simulink model "sm_import_robot_stepfiles"  (R2018b)
settings: Solver=FixedStepAuto  StartTime=0.0  StopTime=50  RelTol=1e-3  EnableMultiTasking=on
undefined symbols (not defined in the file): sigbuilder_block, X, Y, Z
libraries: sm_lib x58, fl_lib x41, nesl_utility x23, Multibody_Multiphysics_Lib x6, elec_lib x3, dspindex x3, arduinolib x2
(part 3 of 3)

== system sm_import_robot_stepfiles/Robot/Gripper/Right Second Finger Link ==
  Base Transform : sm_lib/Frames and Transforms/Rigid Transform  TranslationMethod=Cartesian  TranslationStandardOffset=0  TranslationLengthUnit=cm  TranslationStandardAxis=+Z  TranslationCartesianOffset=[2.1844 -0.91801024484276539 0]  TranslationROffset=0  TranslationROffsetUnits=m  TranslationZOffset=0  TranslationZOffsetUnits=m  TranslationThetaOffset=0  TranslationThetaOffsetUnits=deg  RotationMethod=ArbitraryAxis  RotationAngleUnits=deg  RotationStandardAxis=+Z  RotationAngle=120  RotationArbitraryAxis=[-1 -1 -1]  FollAlignAxisA=+X  BaseAlignAxisA=+Y  FollAlignAxisB=+Y  BaseAlignAxisB=+Z  RotationSequenceAxes=FollowerAxes  RotationSequence=XYX  RotationSequenceAngles=[0 0 0]  RotationSequenceAnglesUnits=deg  RotationMatrix=[1 0 0; 0 1 0; 0 0 1]
  Follower Transform : sm_lib/Frames and Transforms/Rigid Transform  TranslationMethod=Cartesian  TranslationStandardOffset=0  TranslationLengthUnit=cm  TranslationStandardAxis=+Z  TranslationCartesianOffset=[0 0.61321024484276621 0]  TranslationROffset=0  TranslationROffsetUnits=m  TranslationZOffset=0  TranslationZOffsetUnits=m  TranslationThetaOffset=0  TranslationThetaOffsetUnits=deg  RotationMethod=ArbitraryAxis  RotationAngleUnits=deg  RotationStandardAxis=+Z  RotationAngle=120  RotationArbitraryAxis=[1 -1 1]  FollAlignAxisA=+X  BaseAlignAxisA=+Y  FollAlignAxisB=+Y  BaseAlignAxisB=+Z  RotationSequenceAxes=FollowerAxes  RotationSequence=XYX  RotationSequenceAngles=[0 0 0]  RotationSequenceAnglesUnits=deg  RotationMatrix=[1 0 0; 0 1 0; 0 0 1]
  Solid : sm_lib/Body Elements/Solid  InertiaType=CalculateFromGeometry  Mass=0.005347817964666832  MassUnits=kg  CenterOfMass=[1.3095387695944416 0 0]  CenterOfMassUnits=cm  MomentsOfInertia=[0.00062632050801362594 0.0042402045040431545 0.0044495724115703027]  MomentsOfInertiaUnits=kg*cm^2  ProductsOfInertia=[0 0 0]  ProductsOfInertiaUnits=kg*cm^2  BasedOnType=Mass  Density=1000  DensityUnits=kg/(m^3)  DoExposeReferenceFrame=on  SerializedFrames=<Frames/>  GraphicType=FromGeometry  MarkerShape=Sphere  MarkerSize=10  MarkerSizeUnits=m  GraphicVisPropType=SimpleVisualProperties  GraphicDiffuseColor=[1 0 0]  GraphicSpecularColor=[0.5 0.5 0.5 1.0]  GraphicAmbientColor=[0.15 0.15 0.15 1.0]  GraphicEmissiveColor=[0.0 0.0 0.0 1.0]  GraphicShininess=75  GraphicOpacity=1  GeometryShape=FromFile  RectangleSize=[1 1]  RectangleSizeUnits=m  BrickDimensions=[1 1 1]  BrickDimensionUnits=m  CylinderRadius=1  CylinderRadiusUnits=m  CylinderLength=1  CylinderLengthUnits=m  SphereRadius=1  SphereRadiusUnits=m  EllipsoidRadii=[1 1 1]  EllipsoidRadiiUnits=m  ExtrusionCrossSection=[1 1; -1 1; -1 -1; 1 -1]  ExtrusionCrossSectionUnits=m  ExtrusionLength=1  ExtrusionLengthUnits=m  PolygonNumSides=3  PolygonOuterRadius=1  PolygonOuterRadiusUnits=m  ExtGeomFileType=STEP  ExtGeomFileName=sm_srobot_secondfingerlink.step  ExtGeomFileUnits=cm  RevolutionCrossSection=[1 1; 1 -1; 2 -1; 2 1]  RevolutionCrossSectionUnits=m  RevolutionExtent=Full  RevolutionAngle=180  RevolutionAngleUnits=deg
  B : PMIOPort  Side=Left
  F : PMIOPort  Port=2  Side=Right
  connections:
  Solid/RConn1 -- Follower Transform/LConn1 -- Base Transform/LConn1
  Base Transform/RConn1 -- B/RConn1
  Follower Transform/RConn1 -- F/RConn1

== system sm_import_robot_stepfiles/Robot/Gripper Actuation/Gripper Motion ==
  Demux : Demux  Tag=STV Demux  Outputs=1
  FromWs : FromWorkspace  Tag=STV FromWs  VariableName=tuvar  SampleTime=0
      SigBuilderData=|
      | common.afterFinalStr = 'Extrapolate'
      | common.sampleTime = 0
      | dataSet.timeRange = [0 20]
      | dataSet.name = 'Motion'
      | sbobj.Groups.Name = 'Motion'
      | sbobj.Groups.Signals.Name = 'GA'
      | sbobj.Groups.Signals.XData = [0 2.5 4.5 5.5 7.5 12.5 14.5 15.5 17.5 20]
      | sbobj.Groups.Signals.YData = [0 0 0.5 0 0 0 -0.2 -0.2 0 0]
      | sbobj.Groups.TimeRange = [0 20]
  GA : Outport  Tag=STV Outport
  wires:
  Demux/1 -> GA/1
  FromWs/1 -> Demux/1

== system sm_import_robot_stepfiles/Robot/DC Motor1/Counter1/counterA ==
  In1 : Inport
  In2 : Inport  Port=2
  Trigger : TriggerPort  TriggerType=either  VariantControl=Variant  PortDimensions=1
  Add : Sum
  Constant : Constant  SampleTime=-1
  Constant1 : Constant  Value=-1  SampleTime=-1
  Logical Operator : Logic  Operator=XOR  AllPortsSameDT=off  OutDataTypeStr=boolean
  Memory : Memory  InheritSampleTime=on
  Switch : Switch  Criteria=u2 > Threshold
  Out1 : Outport
  wires:
  Constant1/1 -> Switch/3
  Constant/1 -> Switch/1
  Switch/1 -> Add/1
  Logical Operator/1 -> Switch/2
  In2/1 -> Logical Operator/2  "B"
  In1/1 -> Logical Operator/1  "A"
  Add/1 -> Memory/1, Out1/1
  Memory/1 -> Add/2

== system sm_import_robot_stepfiles/Robot/DC Motor1/Counter1/counterB ==
  In1 : Inport
  In2 : Inport  Port=2
  Trigger : TriggerPort  TriggerType=either  VariantControl=Variant  PortDimensions=1
  Add : Sum
  Constant : Constant  Value=-1  SampleTime=-1
  Constant1 : Constant  SampleTime=-1
  Logical Operator : Logic  Operator=XOR  AllPortsSameDT=off  OutDataTypeStr=boolean
  Memory : Memory  InheritSampleTime=on
  Switch : Switch  Criteria=u2 > Threshold
  Out1 : Outport
  wires:
  Memory/1 -> Add/2
  Add/1 -> Out1/1, Memory/1
  In1/1 -> Logical Operator/1  "A"
  In2/1 -> Logical Operator/2  "B"
  Logical Operator/1 -> Switch/2
  Switch/1 -> Add/1
  Constant/1 -> Switch/1
  Constant1/1 -> Switch/3

== system sm_import_robot_stepfiles/Robot/DC Motor2/Counter1/counterA ==
  In1 : Inport
  In2 : Inport  Port=2
  Trigger : TriggerPort  TriggerType=either  VariantControl=Variant  PortDimensions=1
  Add : Sum
  Constant : Constant  SampleTime=-1
  Constant1 : Constant  Value=-1  SampleTime=-1
  Logical Operator : Logic  Operator=XOR  AllPortsSameDT=off  OutDataTypeStr=boolean
  Memory : Memory  InheritSampleTime=on
  Switch : Switch  Criteria=u2 > Threshold
  Out1 : Outport
  wires:
  Memory/1 -> Add/2
  Add/1 -> Out1/1, Memory/1
  In1/1 -> Logical Operator/1  "A"
  In2/1 -> Logical Operator/2  "B"
  Logical Operator/1 -> Switch/2
  Switch/1 -> Add/1
  Constant/1 -> Switch/1
  Constant1/1 -> Switch/3

== system sm_import_robot_stepfiles/Robot/DC Motor2/Counter1/counterB ==
  In1 : Inport
  In2 : Inport  Port=2
  Trigger : TriggerPort  TriggerType=either  VariantControl=Variant  PortDimensions=1
  Add : Sum
  Constant : Constant  Value=-1  SampleTime=-1
  Constant1 : Constant  SampleTime=-1
  Logical Operator : Logic  Operator=XOR  AllPortsSameDT=off  OutDataTypeStr=boolean
  Memory : Memory  InheritSampleTime=on
  Switch : Switch  Criteria=u2 > Threshold
  Out1 : Outport
  wires:
  Constant1/1 -> Switch/3
  Constant/1 -> Switch/1
  Switch/1 -> Add/1
  Logical Operator/1 -> Switch/2
  In2/1 -> Logical Operator/2  "B"
  In1/1 -> Logical Operator/1  "A"
  Add/1 -> Memory/1, Out1/1
  Memory/1 -> Add/2

== system sm_import_robot_stepfiles/Robot/DC Motor3/Counter1/counterA ==
  In1 : Inport
  In2 : Inport  Port=2
  Trigger : TriggerPort  TriggerType=either  VariantControl=Variant  PortDimensions=1
  Add : Sum
  Constant : Constant  SampleTime=-1
  Constant1 : Constant  Value=-1  SampleTime=-1
  Logical Operator : Logic  Operator=XOR  AllPortsSameDT=off  OutDataTypeStr=boolean
  Memory : Memory  InheritSampleTime=on
  Switch : Switch  Criteria=u2 > Threshold
  Out1 : Outport
  wires:
  Memory/1 -> Add/2
  Add/1 -> Out1/1, Memory/1
  In1/1 -> Logical Operator/1  "A"
  In2/1 -> Logical Operator/2  "B"
  Logical Operator/1 -> Switch/2
  Switch/1 -> Add/1
  Constant/1 -> Switch/1
  Constant1/1 -> Switch/3

== system sm_import_robot_stepfiles/Robot/DC Motor3/Counter1/counterB ==
  In1 : Inport
  In2 : Inport  Port=2
  Trigger : TriggerPort  TriggerType=either  VariantControl=Variant  PortDimensions=1
  Add : Sum
  Constant : Constant  Value=-1  SampleTime=-1
  Constant1 : Constant  SampleTime=-1
  Logical Operator : Logic  Operator=XOR  AllPortsSameDT=off  OutDataTypeStr=boolean
  Memory : Memory  InheritSampleTime=on
  Switch : Switch  Criteria=u2 > Threshold
  Out1 : Outport
  wires:
  Constant1/1 -> Switch/3
  Constant/1 -> Switch/1
  Switch/1 -> Add/1
  Logical Operator/1 -> Switch/2
  In2/1 -> Logical Operator/2  "B"
  In1/1 -> Logical Operator/1  "A"
  Add/1 -> Memory/1, Out1/1
  Memory/1 -> Add/2

== system sm_import_robot_stepfiles/Robot/Gripper/Finger Act/Finger Motion ==
  Demux : Demux  Tag=STV Demux  Outputs=2
  FromWs : FromWorkspace  Tag=STV FromWs  VariableName=tuvar  SampleTime=0
      SigBuilderData=|
      | common.afterFinalStr = 'Extrapolate'
      | common.sampleTime = 0
      | dataSet.timeRange = [0 20]
      | dataSet.name = 'Motion'
      | sbobj.Groups.Name = 'Motion'
      | sbobj.Groups.Signals(1).Name = 'FA'
      | sbobj.Groups.Signals(1).XData = [0 4 4.5 4.5 5.5 5.5 6 14.5 15.5 20]
      | sbobj.Groups.Signals(1).YData = [130 130 130 129.8 147 150 150 150 130 130]
      | sbobj.Groups.Signals(2).Name = 'Signal 1'
      | sbobj.Groups.Signals(2).XData = [0 20]
      | sbobj.Groups.Signals(2).YData = [45 45]
      | sbobj.Groups.TimeRange = [0 20]
  FA : Outport  Tag=STV Outport
  Signal 1 : Outport  Tag=STV Outport  Port=2
  wires:
  Demux/1 -> FA/1
  FromWs/1 -> Demux/1
  Demux/2 -> Signal 1/1
